simulink model "ToFile"  (R2015b)
settings: Solver=VariableStepAuto  StartTime=0.0  StopTime=10.0  RelTol=1e-3
libraries: simulink x1
settings Model: Creator=LUBO  LastModifiedBy=LUBO

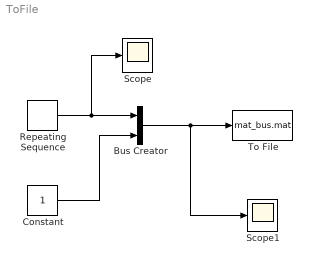
== system ToFile ==
  Bus Creator : BusCreator  Inputs=2
  Constant : Constant
  Repeating Sequence : simulink/Sources/Repeating Sequence  rep_seq_t=[0 1 2]  rep_seq_y=[0 2 0]
  Scope : Scope
  Scope1 : Scope
  To File : ToFile  Filename=mat_bus.mat  SaveFormat=Timeseries
  wires:
  Bus Creator/1 -> Scope1/1, To File/1
  Repeating Sequence/1 -> Scope/1, Bus Creator/1
  Constant/1 -> Bus Creator/2
